simulink model "MPC_gazebo_p2p"  (R2020b)
settings: Solver=FixedStepAuto  StartTime=0.0  StopTime=5  RelTol=1e-3
StopFcn:
  | figHandles = findobj('Type', 'figure');
  | for i = 1: length(figHandles)
  |     if contains(figHandles(i).Name, 'Sign Following Robot', 'IgnoreCase', true)
  |         close(figHandles(i));
  |     end
  | end
  | 
  | clear figHandles;
model workspace (MAT data in the model file):
  SL_ROS_VariableLengthArrays_MaxSizes.CommonInfo.ArrayTruncateAction = 'EmitWarning'
  SL_ROS_VariableLengthArrays_MaxSizes.MsgTypeMap = containers.Map
  SL_ROS_VariableLengthArrays_MaxSizes.MsgTypeMap.serialization.keys = {'gazebo_msgs/ModelStates', 'sensor_msgs/Image'}
  SL_ROS_VariableLengthArrays_MaxSizes.MsgTypeMap.serialization.values{1}(1).PropertyName = 'Name'
  SL_ROS_VariableLengthArrays_MaxSizes.MsgTypeMap.serialization.values{1}(1).DataType = 'std_msgs/String'
  SL_ROS_VariableLengthArrays_MaxSizes.MsgTypeMap.serialization.values{1}(1).MaxLength = 40
  SL_ROS_VariableLengthArrays_MaxSizes.MsgTypeMap.serialization.values{1}(2).PropertyName = 'Pose'
  SL_ROS_VariableLengthArrays_MaxSizes.MsgTypeMap.serialization.values{1}(2).DataType = 'geometry_msgs/Pose'
  SL_ROS_VariableLengthArrays_MaxSizes.MsgTypeMap.serialization.values{1}(2).MaxLength = 40
  SL_ROS_VariableLengthArrays_MaxSizes.MsgTypeMap.serialization.values{1}(3).PropertyName = 'Twist'
  SL_ROS_VariableLengthArrays_MaxSizes.MsgTypeMap.serialization.values{1}(3).DataType = 'geometry_msgs/Twist'
  SL_ROS_VariableLengthArrays_MaxSizes.MsgTypeMap.serialization.values{1}(3).MaxLength = 40
  SL_ROS_VariableLengthArrays_MaxSizes.MsgTypeMap.serialization.values{2}(1).PropertyName = 'Data'
  SL_ROS_VariableLengthArrays_MaxSizes.MsgTypeMap.serialization.values{2}(1).DataType = 'uint8'
  SL_ROS_VariableLengthArrays_MaxSizes.MsgTypeMap.serialization.values{2}(1).MaxLength = 921600
  SL_ROS_VariableLengthArrays_MaxSizes.MsgTypeMap.serialization.values{2}(2).PropertyName = 'Encoding'
  SL_ROS_VariableLengthArrays_MaxSizes.MsgTypeMap.serialization.values{2}(2).DataType = 'uint8'
  SL_ROS_VariableLengthArrays_MaxSizes.MsgTypeMap.serialization.values{2}(2).MaxLength = 128
  SL_ROS_VariableLengthArrays_MaxSizes.MsgTypeMap.serialization.uniformity = 0
  SL_ROS_VariableLengthArrays_MaxSizes.MsgTypeMap.serialization.keyType = 'char'
  SL_ROS_VariableLengthArrays_MaxSizes.MsgTypeMap.serialization.valueType = 'any'
undefined symbols (not defined in the file or in its folder): Angular, Linear
libraries: robotlib x3, robotgazebolib x1, simulink x1
settings Model: Creator=The MathWorks, Inc.  LastModifiedBy=usuario
settings OptimizationCC: EnhancedBackFolding=on  PassReuseOutputArgsThreshold=0  MaxStackSize=64  OptimizeBlockOrder=speed  DifferentSizesBufferReuse=on  OptimizationCustomize=off
settings DebuggingCC: ParameterTunabilityLossMsg=error
settings HardwareCC: ProdBitPerPointer=32  ProdBitPerSizeT=32  ProdBitPerPtrDiffT=32  ProdLargestAtomicFloat=None  ProdIntDivRoundTo=Undefined  ProdEndianess=Unspecified  ProdWordSize=32  ProdHWDeviceType=Generic->Unspecified (assume 32-bit Generic)  UseEmbeddedCoderFeatures=off
settings SFSimCC: MATLABDynamicMemAlloc=off  SimTargetLang=C++
settings RTWCC: Description=Embedded Coder  SystemTargetFile=ert.tlc  HardwareBoard=Robot Operating System (ROS)  TLCOptions="-aInlineSetEventsForThisBaseRateFcn=TLC_FALSE -aSuppressMultiTaskScheduler=TLC_FALSE  -aRateBasedStepFcn=0"  TemplateMakefile=ert_default_tmf  GenerateReport=on  Toolchain=Catkin  LaunchReport=on  TargetLang=C++
settings CodeAppCC: ForceParamTrailComments=on  OperatorAnnotations=on
settings ERTTargetCC: ERTCustomFileBanners=off  SupportContinuousTime=on  SupportNonInlinedSFcns=on  RemoveResetFunc=off  SupportVariableSizeSignals=on  ModelStepFunctionPrototypeControlCompliant=off

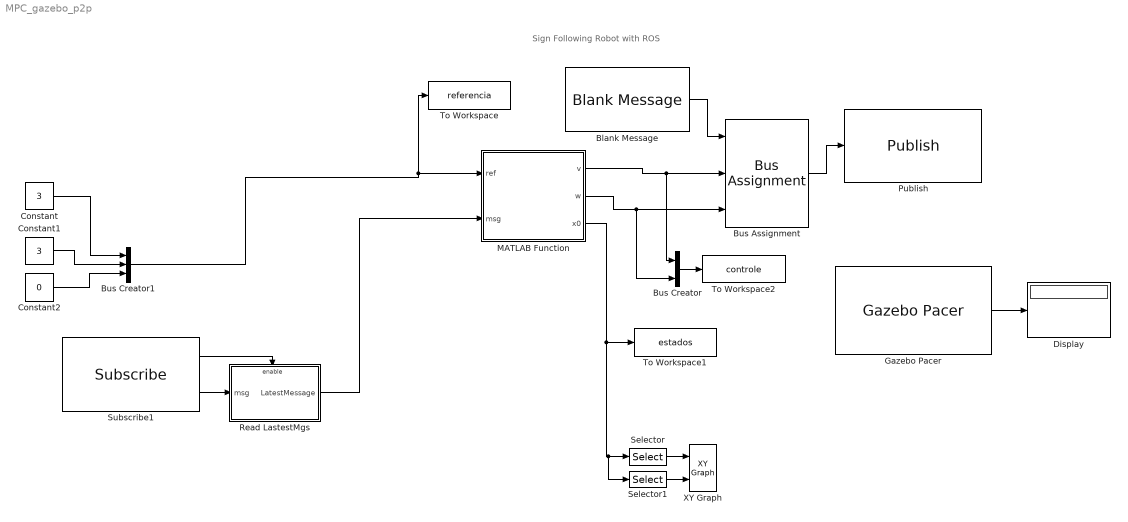
== system MPC_gazebo_p2p ==
  note: Sign Following Robot with ROS
  Blank Message : robotlib/Blank Message  messageClass=Message  entityType=geometry_msgs/Twist  messageType=geometry_msgs/Twist  SampleTime=inf  legacyBusStruct=off
  Bus Assignment : BusAssignment  AssignedSignals=Linear.X,Angular.Z
  Bus Creator : BusCreator  Inputs=2
  Bus Creator1 : BusCreator  Inputs=3
  Constant : Constant  Value=3
  Constant1 : Constant  Value=3
  Constant2 : Constant  Value=0
  Display : Display
  Gazebo Pacer : robotgazebolib/Gazebo Pacer  ResetBehavior=Reset Gazebo simulation time and scene  SampleTime=0.01
      settings: SourceProductBaseCode=RO
  MATLAB Function : MATLAB Function  TreatAsAtomicUnit=on
  Publish : robotlib/Publish  topicSource=Select from ROS network  topic=/husky_velocity_controller/cmd_vel  messageType=geometry_msgs/Twist  legacyBusStruct=off  messageQueueLength=1
  Read LastestMgs : Subsystem  TreatAsAtomicUnit=on
  Selector : Selector  InputPortWidth=3  IndexOptions=Index vector (dialog)  Indices=[1]  OutputSizes=1
  Selector1 : Selector  InputPortWidth=3  IndexOptions=Index vector (dialog)  Indices=[2]  OutputSizes=1
  Subscribe1 : robotlib/Subscribe  topicSource=Select from ROS network  topic=/gazebo/model_states  messageType=gazebo_msgs/ModelStates  SampleTime=-1  legacyBusStruct=off  messageQueueLength=1
  To Workspace : ToWorkspace  VariableName=referencia  SampleTime=-1
  To Workspace1 : ToWorkspace  VariableName=estados  SampleTime=-1
  To Workspace2 : ToWorkspace  VariableName=controle  SampleTime=-1
  XY Graph : simulink/Sinks/XY Graph  xmin=-3  xmax=4  ymin=-1  ymax=8  st=-1
  wires:
  Bus Assignment/1 -> Publish/1
  Blank Message/1 -> Bus Assignment/1
  Gazebo Pacer/1 -> Display/1
  Bus Creator1/1 -> To Workspace/1, MATLAB Function/1(ref)
  MATLAB Function/1(v) -> Bus Creator/1, Bus Assignment/2
  MATLAB Function/2(w) -> Bus Creator/2, Bus Assignment/3
  Selector/1 -> XY Graph/1
  Selector1/1 -> XY Graph/2
  Subscribe1/2 -> Read LastestMgs/1(msg)
  Subscribe1/1 -> Read LastestMgs/Enable
  Read LastestMgs/1(LatestMessage) -> MATLAB Function/2(msg)
  MATLAB Function/3(x0) -> To Workspace1/1, Selector1/1, Selector/1
  Bus Creator/1 -> To Workspace2/1
  Constant/1 -> Bus Creator1/1
  Constant1/1 -> Bus Creator1/2
  Constant2/1 -> Bus Creator1/3

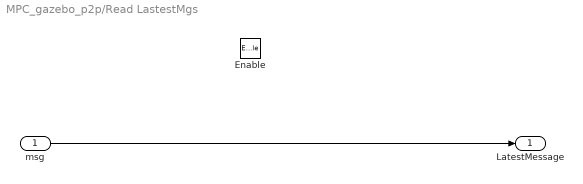
== system MPC_gazebo_p2p/Read LastestMgs ==
  msg : Inport
  Enable : EnablePort
  LatestMessage : Outport
  wires:
  msg/1 -> LatestMessage/1

== matlab function MPC_gazebo_p2p/MATLAB Function ==
  data: ref input; v output; w output; msg input; x0 output
function [v,w,x0] = fcn(ref,msg)



import casadi.*


T = 0.01; %[s]
N = 100; % prediction horizon

v_max = 1; v_min = -v_max;
omega_max = 1.8; omega_min = -omega_max;

x = SX.sym('x'); y = SX.sym('y'); theta = SX.sym('theta');
states = [x;y;theta]; n_states = length(states);

v = SX.sym('v'); omega = SX.sym('omega');
controls = [v;omega]; n_controls = length(controls);
rhs = [v*cos(theta);v*sin(theta);omega]; % system r.h.s

f = Function('f',{states,controls},{rhs}); % nonlinear mapping function f(x,u)
U = SX.sym('U',n_controls,N); % Decision variables (controls)
P = SX.sym('P',n_states + n_states);
% parameters (which include the initial state and the reference state)

X = SX.sym('X',n_states,(N+1));
% A vector that represents the states over the optimization problem.

obj = 0; % Objective function
g = [];  % constraints vector

Q = zeros(3,3); Q(1,1) = 5;Q(2,2) = 5;Q(3,3) = 0.1; % weighing matrices (states)
R = zeros(2,2); R(1,1) = 0.5; R(2,2) = 0.05; % weighing matrices (controls)

st  = X(:,1); % initial state
g = [g;st-P(1:3)]; % initial condition constraints
for k = 1:N
    st = X(:,k);  con = U(:,k);
    obj = obj+(st-P(4:6))'*Q*(st-P(4:6)) + con'*R*con; % calculate obj
    st_next = X(:,k+1);
    f_value = f(st,con);
    st_next_euler = st+ (T*f_value);
    g = [g;st_next-st_next_euler]; % compute constraints
end
% make the decision variable one column  vector
OPT_variables = [reshape(X,3*(N+1),1);reshape(U,2*N,1)];

nlp_prob = struct('f', obj, 'x', OPT_variables, 'g', g, 'p', P);

opts = struct;
opts.ipopt.max_iter = 2000;
opts.ipopt.print_level =0;%0,3
opts.print_time = 0;
opts.ipopt.acceptable_tol =1e-8;
opts.ipopt.acceptable_obj_change_tol = 1e-6;

solver = nlpsol('solver', 'ipopt', nlp_prob,opts);

args = struct;

args.lbg(1:3*(N+1)) = 0;  % -1e-20  % Equality constraints
args.ubg(1:3*(N+1)) = 0;  % 1e-20   % Equality constraints

args.lbx(1:3:3*(N+1),1) = -inf; %state x lower bound
args.ubx(1:3:3*(N+1),1) = inf; %state x upper bound
args.lbx(2:3:3*(N+1),1) = -inf; %state y lower bound
args.ubx(2:3:3*(N+1),1) = inf; %state y upper bound
args.lbx(3:3:3*(N+1),1) = -inf; %state theta lower bound
args.ubx(3:3:3*(N+1),1) = inf; %state theta upper bound

args.lbx(3*(N+1)+1:2:3*(N+1)+2*N,1) = v_min; %v lower bound
args.ubx(3*(N+1)+1:2:3*(N+1)+2*N,1) = v_max; %v upper bound
args.lbx(3*(N+1)+2:2:3*(N+1)+2*N,1) = omega_min; %omega lower bound
args.ubx(3*(N+1)+2:2:3*(N+1)+2*N,1) = omega_max; %omega upper bound
%----------------------------------------------
% ALL OF THE ABOVE IS JUST A PROBLEM SET UP

pos = msg ;
quat = pos.Pose(19, 1).Orientation;
% Tranformação quartenion para Euller
angles = quat2eul([quat.W quat.X quat.Y quat.Z]);
theta = angles(1);
x0 = [pos.Pose(19, 1).Position.X; pos.Pose(19, 1).Position.Y; theta];



xs = ref; % Reference posture.

%xx(:,1) = x0; % xx contains the history of states

u0 = zeros(N,2);        % two control inputs for each robot
X0 = repmat(x0,1,N+1)'; % initialization of the states decision variables

% solução OCP


args.p   = [x0;xs]; % set the values of the parameters vector
% initial value of the optimization variables
args.x0  = [reshape(X0',3*(N+1),1);reshape(u0',2*N,1)];
sol = solver('x0', args.x0, 'lbx', args.lbx, 'ubx', args.ubx,...
    'lbg', args.lbg, 'ubg', args.ubg,'p',args.p);
u = reshape(full(sol.x(3*(N+1)+1:end))',2,N)'; % get controls only from the solution
%xx1(:,1:3,mpciter+1)= reshape(full(sol.x(1:3*(N+1)))',3,N+1)'; % get solution TRAJECTORY
u_cl= u(1,:);



v=u_cl(1);
w=u_cl(2);
